simulink model "second_order_trial"  (Simulink 10.2)
settings: Solver=VariableStepAuto  StartTime=0.0  StopTime=4  RelTol=1e-3
values from neighbouring files (symbols this model uses):
  q0 = [-0.9273 -1.287 1 2.2143]    [generated_traj.mat]
  q0_dot = [0 0 0 0]    [generated_traj.mat]
  Tc = 0.001    [generated_traj.mat]
undefined symbols (not defined in the file or in its folder): DiscIntNeverNeededParam
settings Model: Creator=RAJESH ANAND  LastModifiedBy=Megha Veerendra
settings DataIOCC: SaveFormat=Dataset  SignalLoggingSaveFormat=Dataset  ReturnWorkspaceOutputs=on
settings OptimizationCC: LifeSpan=auto
settings DebuggingCC: UnderspecifiedInitializationDetection=Simplified  MergeDetectMultiDrivingBlocksExec=error  FcnCallInpInsideContextMsg=error  SFUnexpectedBacktrackingDiag=error  SFNoUnconditionalDefaultTransitionDiag=error  SFExecutionAtInitializationDiag=warning
settings HardwareCC: ProdBitPerPointer=64  ProdBitPerSizeT=64  ProdBitPerPtrDiffT=64  ProdLargestAtomicFloat=Float  ProdIntDivRoundTo=Zero  ProdEndianess=LittleEndian  ProdWordSize=64  ProdHWDeviceType=Intel->x86-64 (Windows64)
settings ModelReferenceCC: PropagateSignalLabelsOutOfModel=on
settings SFSimCC: SimUseLocalCustomCode=on
settings RTWCC: RTWUseLocalCustomCode=on
settings CodeAppCC: StateflowObjectComments=off
settings GRTTargetCC: TargetLangStandard=C99 (ISO)  CombineOutputUpdateFcns=on  GRTInterface=off
settings ConfigComp: CovMetricSettings=dwe  CovSaveCumulativeToWorkspaceVar=off  CovSaveSingleToWorkspaceVar=off  CovExternalEMLEnable=on

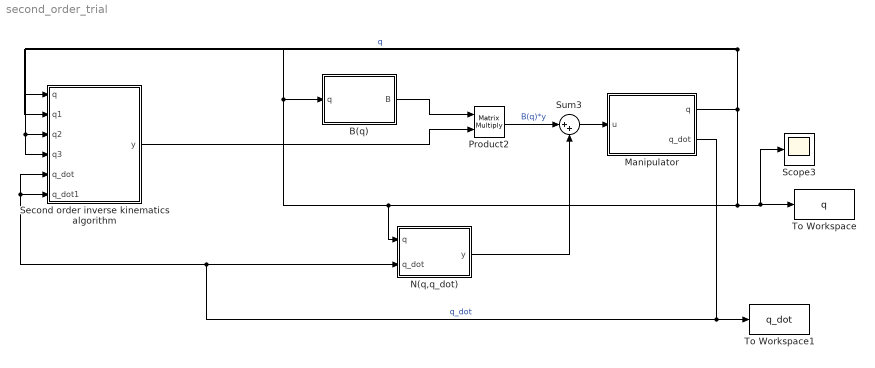
== system second_order_trial ==
  B(q) : MATLAB Function  TreatAsAtomicUnit=on
  Manipulator : Subsystem
  N(q,q_dot) : MATLAB Function  TreatAsAtomicUnit=on
  Product2 : Product  Multiplication=Matrix(*)
  Scope3 : Scope
  Second order inverse kinematics algorithm : Subsystem
  Sum3 : Sum  Inputs=|++
  To Workspace : ToWorkspace  VariableName=q  SampleTime=Tc
      settings: Save2DSignal=2-D array (concatenate along first dimension)
  To Workspace1 : ToWorkspace  VariableName=q_dot  SampleTime=Tc
      settings: Save2DSignal=2-D array (concatenate along first dimension)
  wires:
  Product2/1 -> Sum3/1  "B(q)*y"
  B(q)/1(B) -> Product2/1
  N(q,q_dot)/1(y) -> Sum3/2
  Manipulator/1(q) -> Second order inverse kinematics algorithm/3(q2), Second order inverse kinematics algorithm/4(q3), Second order inverse kinematics algorithm/2(q1), To Workspace/1, Scope3/1, Second order inverse kinematics algorithm/1(q), B(q)/1(q), N(q,q_dot)/1(q)  "q"
  Manipulator/2(q_dot) -> Second order inverse kinematics algorithm/5(q_dot), Second order inverse kinematics algorithm/6(q_dot1), N(q,q_dot)/2(q_dot), To Workspace1/1  "q_dot"
  Sum3/1 -> Manipulator/1(u)
  Second order inverse kinematics algorithm/1(y) -> Product2/2

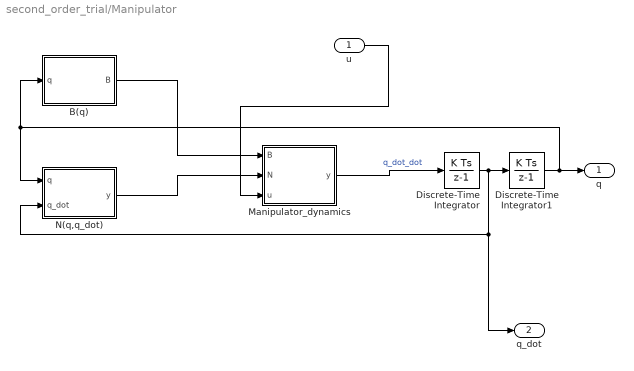
== system second_order_trial/Manipulator ==
  u : Inport
  B(q) : MATLAB Function  TreatAsAtomicUnit=on
  Discrete-Time Integrator : DiscreteIntegrator  InitialCondition=q0_dot  SampleTime=Tc  ICPrevOutput=DiscIntNeverNeededParam  ICPrevScaledInput=DiscIntNeverNeededParam
  Discrete-Time Integrator1 : DiscreteIntegrator  InitialCondition=q0  SampleTime=Tc  ICPrevOutput=DiscIntNeverNeededParam  ICPrevScaledInput=DiscIntNeverNeededParam
  Manipulator_dynamics : MATLAB Function  TreatAsAtomicUnit=on
  N(q,q_dot) : MATLAB Function  TreatAsAtomicUnit=on
  q : Outport
  q_dot : Outport  Port=2
  wires:
  Discrete-Time Integrator/1 -> N(q,q_dot)/2(q_dot), q_dot/1, Discrete-Time Integrator1/1
  Manipulator_dynamics/1(y) -> Discrete-Time Integrator/1  "q_dot_dot"
  Discrete-Time Integrator1/1 -> N(q,q_dot)/1(q), B(q)/1(q), q/1
  u/1 -> Manipulator_dynamics/3(u)
  N(q,q_dot)/1(y) -> Manipulator_dynamics/2(N)
  B(q)/1(B) -> Manipulator_dynamics/1(B)

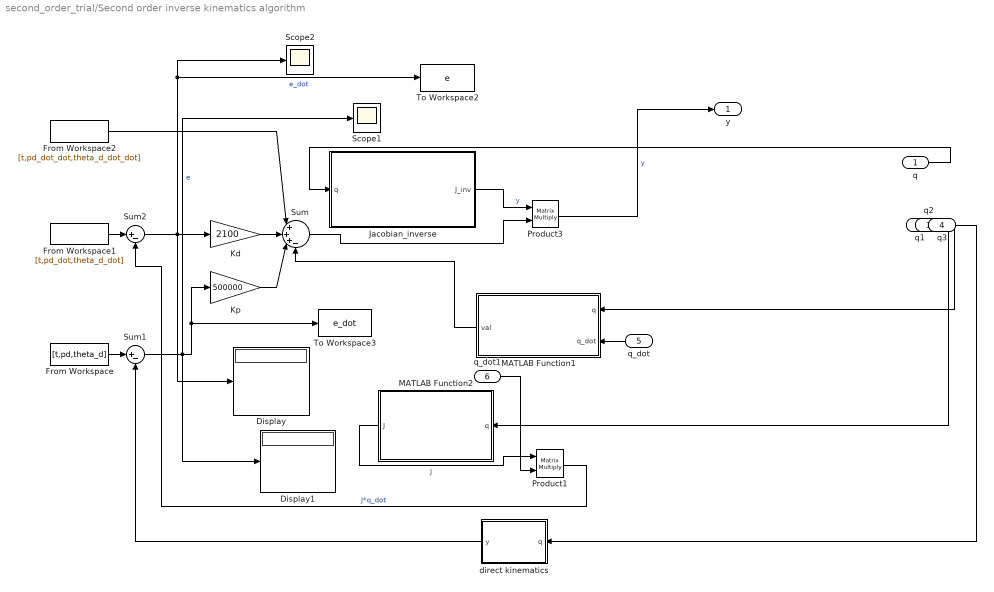
== system second_order_trial/Second order inverse kinematics algorithm ==
  q : Inport
  q1 : Inport  Port=2
  q2 : Inport  Port=3
  q3 : Inport  Port=4
  q_dot : Inport  Port=5
  q_dot1 : Inport  Port=6
  Display : Display
  Display1 : Display
  From Workspace : FromWorkspace  VariableName=[t,pd,theta_d]  SampleTime=Tc
  From Workspace1 : FromWorkspace  VariableName=[t,pd_dot,theta_d_dot]  SampleTime=Tc
  From Workspace2 : FromWorkspace  VariableName=[t,pd_dot_dot,theta_d_dot_dot]  SampleTime=Tc
  Jacobian_inverse : MATLAB Function  TreatAsAtomicUnit=on
  Kd : Gain  Gain=2100
  Kp : Gain  Gain=500000
  MATLAB Function1 : MATLAB Function  TreatAsAtomicUnit=on
  MATLAB Function2 : MATLAB Function  TreatAsAtomicUnit=on
  Product1 : Product  Multiplication=Matrix(*)
  Product3 : Product  Multiplication=Matrix(*)
  Scope1 : Scope
  Scope2 : Scope
  Sum : Sum  Inputs=|+++-
  Sum1 : Sum  Inputs=|+-
  Sum2 : Sum  Inputs=|+-
  To Workspace2 : ToWorkspace  VariableName=e  SampleTime=Tc
      settings: Save2DSignal=2-D array (concatenate along first dimension)
  To Workspace3 : ToWorkspace  VariableName=e_dot  SampleTime=Tc
      settings: Save2DSignal=2-D array (concatenate along first dimension)
  direct kinematics : MATLAB Function  TreatAsAtomicUnit=on
  y : Outport
  wires:
  Product1/1 -> Sum2/2  "J*q_dot"
  direct kinematics/1(y) -> Sum1/2
  Kp/1 -> Sum/3
  Sum1/1 -> Display1/1, Scope1/1, Kp/1, To Workspace3/1  "e"
  q_dot/1 -> MATLAB Function1/2(q_dot)
  Sum2/1 -> Display/1, Kd/1, To Workspace2/1, Scope2/1  "e_dot"
  Jacobian_inverse/1(J_inv) -> Product3/1  "y"
  MATLAB Function2/1(J) -> Product1/1  "J"
  q/1 -> Jacobian_inverse/1(q)
  From Workspace/1 -> Sum1/1
  From Workspace1/1 -> Sum2/1
  MATLAB Function1/1(val) -> Sum/4
  Kd/1 -> Sum/2
  From Workspace2/1 -> Sum/1
  Sum/1 -> Product3/2
  q_dot1/1 -> Product1/2
  q1/1 -> MATLAB Function1/1(q)
  q2/1 -> MATLAB Function2/1(q)
  Product3/1 -> y/1  "y"
  q3/1 -> direct kinematics/1(q)

== matlab function Second order inverse kinematics algorithm/Jacobian_inverse ==
  data: q input double; J_inv output double
function J_inv = Jacobian_Inverse(q)
J_inv = Jacobian_Inverse(q);

end

== matlab function Second order inverse kinematics algorithm/direct kinematics ==
  data: q input double; y output double
function y = direct_kin(q)



y = direct_kin(q);
end

== matlab function Second order inverse kinematics algorithm/MATLAB Function1 ==
  data: q input double; val output double; q_dot input double
function val = Jacobian_dot(q,q_dot)

t1 = q(1,1);
t2 = q(2,1);
d3 = q(3,1);
t4 = q(4,1);

t1_dot = q_dot(1,1);
t2_dot = q_dot(2,1);
d3_dot = q_dot(3,1);
t4_dot = q_dot(4,1);

J11 = -0.5*cos(t1)*(t1_dot) -0.5*cos(t1+t2)*(t1_dot+t2_dot);
J12 = -0.5*cos(t1+t2)*(t1_dot+t2_dot);
J13 = 0;
J14 = 0;
J21 = -0.5*sin(t1)*(t1_dot) - 0.5*sin(t1+t2)*(t1_dot+t2_dot);
J22 = -0.5*sin(t1+t2)*(t1_dot+t2_dot);
J23 = 0;
J24 = 0;
J31 = 0;
J32 = 0;
J33 = 0;
J34 = 0;
J41 = 0;
J42 = 0;
J43 = 0;
J44 = 0;

JacobianDot = [J11 J12 J13 J14;
               J21 J22 J23 J24;
               J31 J32 J33 J34;
               J41 J42 J43 J44];
        
val = JacobianDot * q_dot;

== matlab function Second order inverse kinematics algorithm/MATLAB Function2 ==
  data: q input double; J output double
function J = Jacobian(q)


        
J = Jacobian(q);
end

== matlab function B(q) ==
  data: q input double; B output double
function B = b(q)

B = B_q(q);
end

== matlab function N(q,q_dot) ==
  data: q input double; y output double; q_dot input double
function y = n(q,q_dot)
 
y = N_q_q_dot(q,q_dot);
end

== matlab function Manipulator/Manipulator_dynamics ==
  data: B input double; N input double; u input double; y output double
function y = Manipulator(B,N,u)
  
y = inv(B)*(u-N);

== matlab function Manipulator/N(q,q_dot) ==
  data: q input double; y output double; q_dot input double
function y = n(q,q_dot)
F = [0.0001,0,0,0;0,0.0001,0,0;0,0,0.01,0;0,0,0,0.005];
f = F*q_dot;
y = N_q_q_dot(q,q_dot)+f;
end

== matlab function Manipulator/B(q) ==
  data: q input double; B output double
function B = b(q)

B = B_q(q);
end
